simulink model "model242"  (R2024b)
settings: Solver=VariableStepAuto  StartTime=0.0  StopTime=10.0  RelTol=1e-3
settings Model: Creator=Xist  LastModifiedBy=Xist

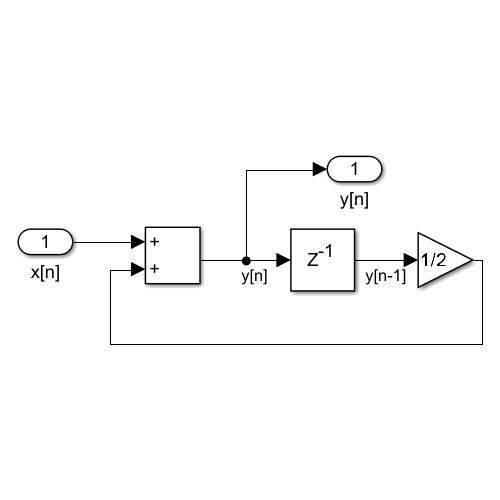
[thumbnail: Simulink's stored preview of the top-level diagram]
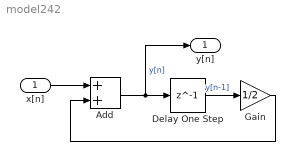
== system model242 ==
  x[n] : Inport
  Add : Sum
  Delay One Step : Delay  DelayLength=1
  Gain : Gain  Gain=1/2
  y[n] : Outport
  wires:
  x[n]/1 -> Add/1
  Delay One Step/1 -> Gain/1  "y[n-1]"
  Add/1 -> Delay One Step/1, y[n]/1  "y[n]"
  Gain/1 -> Add/2
